simulink model "Cascata"  (R2019a)
settings: Solver=VariableStepAuto  StartTime=0.0  StopTime=20  RelTol=1e-3
settings Model: Creator=Usuario  LastModifiedBy=Usuario

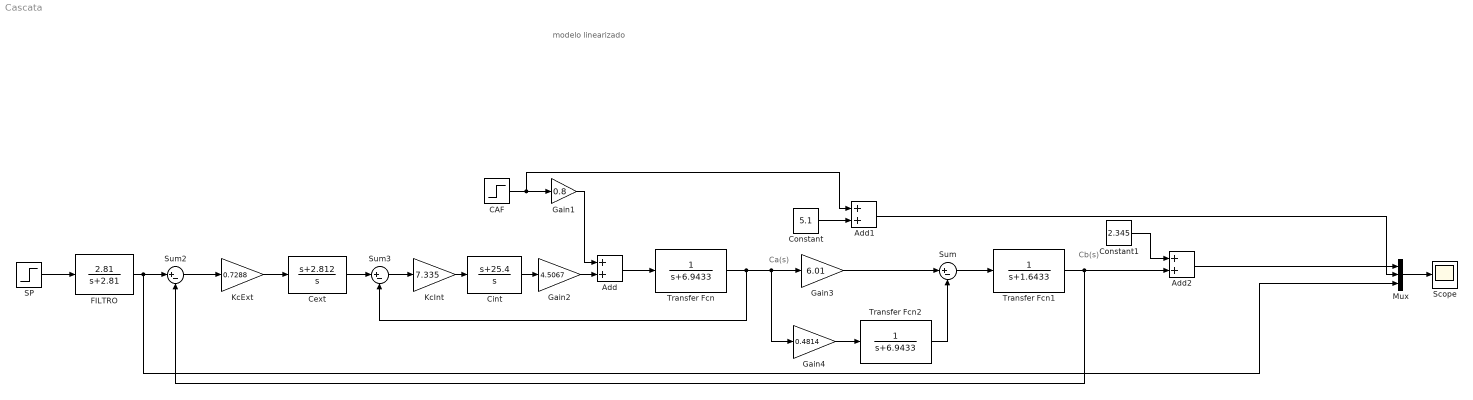
== system Cascata ==
  note: Cb(s)
  note: Ca(s)
  note: modelo linearizado
  Add : Sum
  Add1 : Sum
  Add2 : Sum
  CAF : Step  Time=10  SampleTime=0.01
  "Cext " : TransferFcn  Numerator=[1 2.812]  Denominator=[1 0]
  Cint : TransferFcn  Numerator=[1 25.4]  Denominator=[1 0]
  Constant : Constant  Value=5.1
  Constant1 : Constant  Value=2.345
  "FILTRO " : TransferFcn  Numerator=[2.81]  Denominator=[1 2.81]
  Gain1 : Gain  Gain=0.8
  Gain2 : Gain  Gain=4.5067
  Gain3 : Gain  Gain=6.01
  Gain4 : Gain  Gain=0.4814
  "KcExt " : Gain  Gain=0.7288
  "KcInt " : Gain  Gain=7.335
  Mux : Mux  Inputs=3
  SP : Step  Time=5  After=0.1  SampleTime=0.01
  Scope : Scope
  Sum : Sum  Inputs=|+-
  Sum2 : Sum  Inputs=|+-
  Sum3 : Sum  Inputs=|+-
  Transfer Fcn : TransferFcn  Denominator=[1 6.9433]
  Transfer Fcn1 : TransferFcn  Denominator=[1 1.6433]
  Transfer Fcn2 : TransferFcn  Denominator=[1 6.9433]
  wires:
  Sum/1 -> Transfer Fcn1/1
  Transfer Fcn/1 -> Gain4/1, Gain3/1, Sum3/2
  Add/1 -> Transfer Fcn/1
  "KcExt "/1 -> "Cext "/1
  CAF/1 -> Add1/1, Gain1/1
  Sum2/1 -> "KcExt "/1
  Transfer Fcn1/1 -> Add2/2, Sum2/2
  "FILTRO "/1 -> Mux/3, Sum2/1
  SP/1 -> "FILTRO "/1
  "Cext "/1 -> Sum3/1
  Cint/1 -> Gain2/1
  Gain2/1 -> Add/2
  Gain1/1 -> Add/1
  Gain3/1 -> Sum/1
  Gain4/1 -> Transfer Fcn2/1
  Transfer Fcn2/1 -> Sum/2
  Sum3/1 -> "KcInt "/1
  "KcInt "/1 -> Cint/1
  Mux/1 -> Scope/1
  Constant/1 -> Add1/2
  Add1/1 -> Mux/2
  Constant1/1 -> Add2/1
  Add2/1 -> Mux/1
